simulink library "reorder_library"  (Simulink 6.2)
values from neighbouring files (symbols this model uses):
  bigColBits = 0    [address_gen_dram_mask.m]
  bigRowBits = log2(bigRowLength)    [address_gen_dram_mask.m]
  smallColBits = 0    [address_gen_dram_mask.m]
  smallRowBits = log2(smallRowLength)    [address_gen_dram_mask.m]
undefined symbols (not defined in the file or in its folder): n_bits, order, order_bits
libraries: xbsIndex_r3 x167, fft_library x3, reorder_library x3, xps_library x2, delay_lib x2, simulink x1
settings Model: LastModifiedBy=hchen05

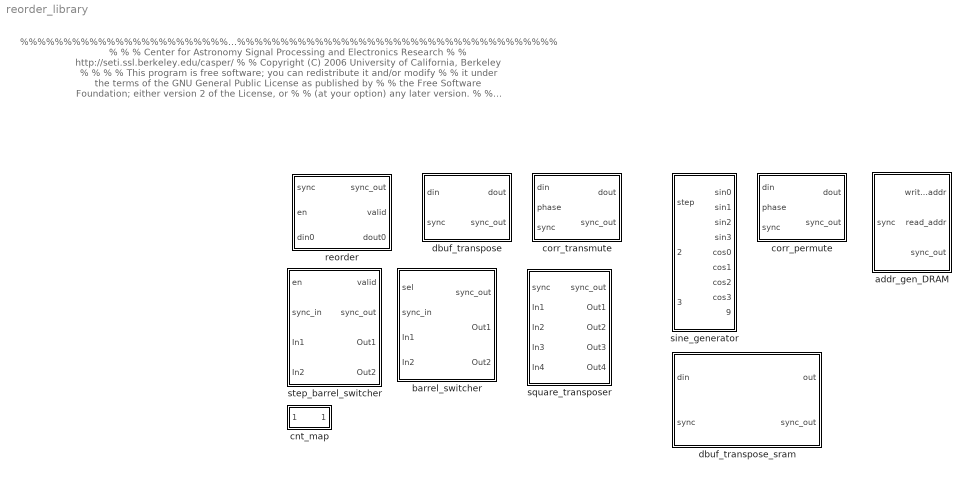
== system reorder_library ==
  note: %%%%%%%%%%%%%%%%%%%%%%%%%%%%%%%%%%%%%%%%%%%%%%%%%%%%%%%%%%%%%%%%%%%%%%%%%%%%%%%
      | %                                                                             %
      | %   Center for Astronomy Signal Processing and Electronics Research           %
      | %   http://seti.ssl.berkeley.edu/casper/                                      %
      | %   Copyright (C) 2006 University of California, Berkeley                     %
      | %                                                                             %
      | %   This program is free software; you can redistribute it and/or modify      %
      | %   it under the terms of the GNU General Public License as published by      %
      | %   the Free Software Foundation; either version 2 of the License, or         %
      | %   (at your option) any later version.                                       %
      | %                                                                             %
      | %   This program is distributed in the hope that it will be useful,           %
      | %   but WITHOUT ANY WARRANTY; without even the implied warranty of            %
      | %   MERCHANTABILITY or FITNESS FOR A PARTICULAR PURPOSE.  See the             %
      | %   GNU General Public License for more details.                              %
      | %                                                                             %
      | %   You should have received a copy of the GNU General Public License along   %
      | %   with this program; if not, write to the Free Software Foundation, Inc.,   %
      | %   51 Franklin Street, Fifth Floor, Boston, MA 02110-1301 USA.               %
      | %                                                                             %
      | %%%%%%%%%%%%%%%%%%%%%%%%%%%%%%%%%%%%%%%%%%%%%%%%%%%%%%%%%%%%%%%%%%%%%%%%%%%%%%%
  addr_gen_DRAM : Subsystem  mask{numSpecs=512, length=1024}
      mask prompts: numSpecs "Number of Spectrums?"; length "Lenght of Spectrum?"
      mask init:
      | address_gen_dram_mask_temp;
  barrel_switcher : Subsystem  mask{n_inputs=1}
      mask prompts: n_inputs "Number of Inputs: (2^?)"
      mask init:
      | barrel_switcher_mask;
  cnt_map : Subsystem  mask(cnt_map){n_bits=2, map=[0 2 1 3], latency=0, old_map=[0 2 1 3]}
      mask prompts: n_bits "Number of bits:"; map "Output order:"; old_map "old map"
      mask init:
      | cnt_map_mask;
  corr_permute : Subsystem  mask{ant_bits=4, add_latency=2, bram_latency=2}
      mask prompts: ant_bits "Number of Antennas: (2^?)"; add_latency "Add Latency"; bram_latency "BRAM Latency"
      mask init:
      | Rows = ant_bits;
  corr_transmute : Subsystem  mask{Rows=2, Cols=3, bram_latency=2, add_latency=2, ant_bits=3}
      mask prompts: Rows "Rows of Matrix (data written in): (2^?)"; Cols "Cols of Matrix (data read out): (2^?)"; bram_latency "BRAM Latency"; add_latency "Add Latency"; ant_bits "Number of Antennas: (2^?)"
  dbuf_transpose : Subsystem  mask{Rows=2, Cols=3, bram_latency=2}
      mask prompts: Rows "Rows of Matrix (data written in): (2^?)"; Cols "Cols of Matrix (data read out): (2^?)"; bram_latency "BRAM Latency"
  dbuf_transpose_sram : Subsystem  mask{length=256, numSpecs=256}
      mask prompts: length "Length of Spectrums"; numSpecs "Number of Spectrums"
      mask help: Sram transpose using double buffering method, maximum size is 256 spectrums by 2048 channels!!
  reorder : Subsystem  mask{map=[0 2 1 3], n_inputs=1, bram_latency=2, map_latency=1}
      mask prompts: map "Output Order:"; n_inputs "Number of inputs"; bram_latency "BRAM Latency"; map_latency "Map Latency"
      mask init:
      | reorder_mask;
  sine_generator : Subsystem  mask{bits=8}
      mask prompts: bits "bitwidth?"
      mask help: Outputs sine and cosine sequences with variable frequency depending on the value of step. If value of step is greater or equal to 2^24 and multiple of 4 then sin0 to sin3 (cos0 to cos3) are consecutive samples of the same sine/cos wave!
  square_transposer : Subsystem  mask{n_inputs=2}
      mask prompts: n_inputs "Number of inputs (2^?):"
      mask init:
      | square_transposer_mask;
  step_barrel_switcher : Subsystem  mask{n_inputs=1, step_dir=Up}
      mask prompts: n_inputs "Number of Inputs: (2^?)"; step_dir "Step Direction"
      mask init:
      | step_barrel_switcher_mask;
      mask StyleString: edit,popup(Up|Down)

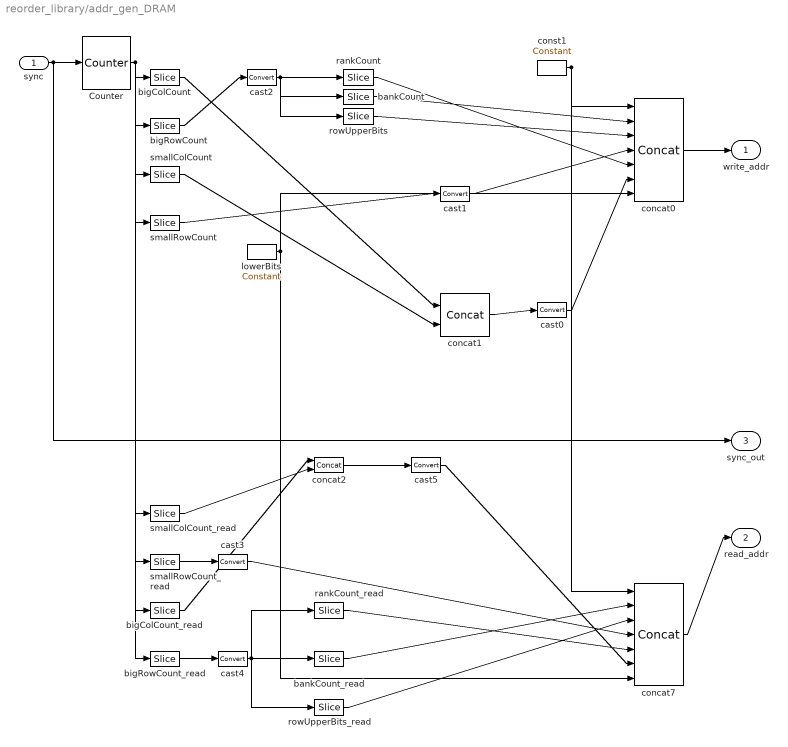
== system reorder_library/addr_gen_DRAM ==
  sync : Inport  Port=1  LatchInput=off
  Counter : xbsIndex_r3/Counter  cnt_type=Free Running  n_bits=counterBitwidth  bin_pt=0  arith_type=Unsigned  start_count=0  cnt_to=Inf  cnt_by_val=1  operation=Up  explicit_period=off  period=1  load_pin=off  rst=on  en=off  dbl_ovrd=off  show_param=off  use_rpm=on  gen_core=off
      settings: xl_area=[0, 0, 0, 0, 0, 0, 0]
  bankCount : xbsIndex_r3/Slice  mode=Upper Bit Location + Width  nbits=2  bit1=-1  base1=MSB of Input  bit0=0  base0=LSB of Input  boolean_output=off  explicit_period=off  period=1  dbl_ovrd=off
  bankCount_read : xbsIndex_r3/Slice  mode=Upper Bit Location + Width  nbits=2  bit1=-1  base1=MSB of Input  bit0=0  base0=LSB of Input  boolean_output=off  explicit_period=off  period=1  dbl_ovrd=off
  bigColCount : xbsIndex_r3/Slice  mode=Lower Bit Location + Width  nbits=bigColBits  bit1=0  base1=MSB of Input  bit0=smallRowBits+smallColBits+8  base0=LSB of Input  boolean_output=off  explicit_period=off  period=1  dbl_ovrd=off
  bigColCount_read : xbsIndex_r3/Slice  mode=Lower Bit Location + Width  nbits=bigColBits  bit1=0  base1=MSB of Input  bit0=bigRowBits  base0=LSB of Input  boolean_output=off  explicit_period=off  period=1  dbl_ovrd=off
  bigRowCount : xbsIndex_r3/Slice  mode=Lower Bit Location + Width  nbits=bigRowBits  bit1=0  base1=MSB of Input  bit0=smallRowBits+smallColBits  base0=LSB of Input  boolean_output=off  explicit_period=off  period=1  dbl_ovrd=off
  bigRowCount_read : xbsIndex_r3/Slice  mode=Lower Bit Location + Width  nbits=bigRowBits  bit1=0  base1=MSB of Input  bit0=0  base0=LSB of Input  boolean_output=off  explicit_period=off  period=1  dbl_ovrd=off
  cast0 : xbsIndex_r3/Convert  arith_type=Unsigned  n_bits=10  bin_pt=0  quantization=Truncate  overflow=Wrap  latency=0  explicit_period=off  period=1  dbl_ovrd=off  show_param=off  inserted_by_tool=off  pipeline=off
      settings: xl_area=[0, 0, 0, 0, 0, 0, 0]
  cast1 : xbsIndex_r3/Convert  arith_type=Unsigned  n_bits=9  bin_pt=0  quantization=Truncate  overflow=Wrap  latency=0  explicit_period=off  period=1  dbl_ovrd=off  show_param=off  inserted_by_tool=off  pipeline=off
      settings: xl_area=[0, 0, 0, 0, 0, 0, 0]
  cast2 : xbsIndex_r3/Convert  arith_type=Unsigned  n_bits=8  bin_pt=0  quantization=Truncate  overflow=Wrap  latency=0  explicit_period=off  period=1  dbl_ovrd=off  show_param=off  inserted_by_tool=off  pipeline=off
      settings: xl_area=[0, 0, 0, 0, 0, 0, 0]
  cast3 : xbsIndex_r3/Convert  arith_type=Unsigned  n_bits=9  bin_pt=0  quantization=Truncate  overflow=Wrap  latency=0  explicit_period=off  period=1  dbl_ovrd=off  show_param=off  inserted_by_tool=off  pipeline=off
      settings: xl_area=[0, 0, 0, 0, 0, 0, 0]
  cast4 : xbsIndex_r3/Convert  arith_type=Unsigned  n_bits=8  bin_pt=0  quantization=Truncate  overflow=Wrap  latency=0  explicit_period=off  period=1  dbl_ovrd=off  show_param=off  inserted_by_tool=off  pipeline=off
      settings: xl_area=[0, 0, 0, 0, 0, 0, 0]
  cast5 : xbsIndex_r3/Convert  arith_type=Unsigned  n_bits=10  bin_pt=0  quantization=Truncate  overflow=Wrap  latency=0  explicit_period=off  period=1  dbl_ovrd=off  show_param=off  inserted_by_tool=off  pipeline=off
      settings: xl_area=[0, 0, 0, 0, 0, 0, 0]
  concat0 : xbsIndex_r3/Concat  num_inputs=7  explicit_period=off  period=1  dbl_ovrd=off
  concat1 : xbsIndex_r3/Concat  num_inputs=2  explicit_period=off  period=1  dbl_ovrd=off
  concat2 : xbsIndex_r3/Concat  num_inputs=2  explicit_period=off  period=1  dbl_ovrd=off
  concat7 : xbsIndex_r3/Concat  num_inputs=7  explicit_period=off  period=1  dbl_ovrd=off
  const1 : xbsIndex_r3/Constant  const=0  equ=P=C  arith_type=Unsigned  n_bits=2  bin_pt=0  opselect=C  inp2=PCIN>>17  opr=+  inp1=P  carry=CIN  iostate=0  explicit_period=on  period=1  dbl_ovrd=off
  lowerBits : xbsIndex_r3/Constant  const=0  equ=P=C  arith_type=Unsigned  n_bits=3  bin_pt=0  opselect=C  inp2=PCIN>>17  opr=+  inp1=P  carry=CIN  iostate=0  explicit_period=on  period=1  dbl_ovrd=off
  rankCount : xbsIndex_r3/Slice  mode=Upper Bit Location + Width  nbits=1  bit1=0  base1=MSB of Input  bit0=0  base0=LSB of Input  boolean_output=off  explicit_period=off  period=1  dbl_ovrd=off
  rankCount_read : xbsIndex_r3/Slice  mode=Upper Bit Location + Width  nbits=1  bit1=0  base1=MSB of Input  bit0=0  base0=LSB of Input  boolean_output=off  explicit_period=off  period=1  dbl_ovrd=off
  rowUpperBits : xbsIndex_r3/Slice  mode=Lower Bit Location + Width  nbits=5  bit1=0  base1=MSB of Input  bit0=0  base0=LSB of Input  boolean_output=off  explicit_period=off  period=1  dbl_ovrd=off
  rowUpperBits_read : xbsIndex_r3/Slice  mode=Lower Bit Location + Width  nbits=5  bit1=0  base1=MSB of Input  bit0=0  base0=LSB of Input  boolean_output=off  explicit_period=off  period=1  dbl_ovrd=off
  smallColCount : xbsIndex_r3/Slice  mode=Lower Bit Location + Width  nbits=smallColBits  bit1=0  base1=MSB of Input  bit0=smallRowBits  base0=LSB of Input  boolean_output=off  explicit_period=off  period=1  dbl_ovrd=off
  smallColCount_read : xbsIndex_r3/Slice  mode=Lower Bit Location + Width  nbits=smallColBits  bit1=0  base1=MSB of Input  bit0=bigRowBits+bigColBits+smallRowBits  base0=LSB of Input  boolean_output=off  explicit_period=off  period=1  dbl_ovrd=off
  smallRowCount : xbsIndex_r3/Slice  mode=Lower Bit Location + Width  nbits=smallRowBits  bit1=0  base1=MSB of Input  bit0=0  base0=LSB of Input  boolean_output=off  explicit_period=off  period=1  dbl_ovrd=off
  smallRowCount_read : xbsIndex_r3/Slice  mode=Lower Bit Location + Width  nbits=smallRowBits  bit1=0  base1=MSB of Input  bit0=bigRowBits+bigColBits  base0=LSB of Input  boolean_output=off  explicit_period=off  period=1  dbl_ovrd=off
  write_addr : Outport
  read_addr : Outport  Port=2
  sync_out : Outport  Port=3
  wires:
  Counter/1 -> bigColCount/1, smallColCount/1, bigColCount_read/1, smallColCount_read/1, smallRowCount/1, bigRowCount/1, smallRowCount_read/1, bigRowCount_read/1
  bigColCount/1 -> concat1/1
  smallColCount/1 -> concat1/2
  concat1/1 -> cast0/1
  smallColCount_read/1 -> concat2/2
  bigColCount_read/1 -> concat2/1
  concat2/1 -> cast5/1
  sync/1 -> Counter/1, sync_out/1
  lowerBits/1 -> concat0/7, concat7/7
  cast0/1 -> concat0/6
  cast5/1 -> concat7/6
  rankCount/1 -> concat0/5
  rankCount_read/1 -> concat7/5
  cast1/1 -> concat0/4
  cast3/1 -> concat7/4
  smallRowCount/1 -> cast1/1
  rowUpperBits/1 -> concat0/3
  rowUpperBits_read/1 -> concat7/3
  bankCount/1 -> concat0/2
  bankCount_read/1 -> concat7/2
  const1/1 -> concat0/1, concat7/1
  bigRowCount/1 -> cast2/1
  cast2/1 -> bankCount/1, rankCount/1, rowUpperBits/1
  smallRowCount_read/1 -> cast3/1
  bigRowCount_read/1 -> cast4/1
  cast4/1 -> rankCount_read/1, bankCount_read/1, rowUpperBits_read/1
  concat0/1 -> write_addr/1
  concat7/1 -> read_addr/1

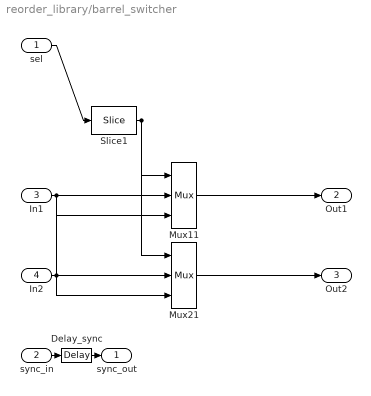
== system reorder_library/barrel_switcher ==
  sel : Inport  Port=1  LatchInput=off
  sync_in : Inport  Port=2  LatchInput=off
  In1 : Inport  Port=3  LatchInput=off
  In2 : Inport  Port=4  LatchInput=off
  Delay_sync : xbsIndex_r3/Delay  latency=1  reg_retiming=off  explicit_period=off  period=1  en=off  accept_only_valid=off  init_zero=on  dbl_ovrd=off  show_param=off
      settings: xl_area=[0, 0, 0, 0, 0, 0, 0]
  Mux11 : xbsIndex_r3/Mux  inputs=2  precision=Full  arith_type="Signed  (2's comp)"  n_bits=8  bin_pt=2  quantization=Truncate  overflow=Wrap  latency=1  explicit_period=off  period=1  en=off  dbl_ovrd=off  show_param=off  mux_type=off  use_rpm=off  gen_core=off
      settings: xl_area=[0, 0, 0, 0, 0, 0, 0]
  Mux21 : xbsIndex_r3/Mux  inputs=2  precision=Full  arith_type="Signed  (2's comp)"  n_bits=8  bin_pt=2  quantization=Truncate  overflow=Wrap  latency=1  explicit_period=off  period=1  en=off  dbl_ovrd=off  show_param=off  mux_type=off  use_rpm=off  gen_core=off
      settings: xl_area=[0, 0, 0, 0, 0, 0, 0]
  Slice1 : xbsIndex_r3/Slice  mode=Upper Bit Location + Width  nbits=1  bit1=-0  base1=MSB of Input  bit0=0  base0=LSB of Input  boolean_output=off  explicit_period=off  period=1  dbl_ovrd=off
  sync_out : Outport
  Out1 : Outport  Port=2
  Out2 : Outport  Port=3
  wires:
  sync_in/1 -> Delay_sync/1
  Delay_sync/1 -> sync_out/1
  sel/1 -> Slice1/1
  Slice1/1 -> Mux11/1, Mux21/1
  In1/1 -> Mux11/2, Mux21/3
  Mux11/1 -> Out1/1
  In2/1 -> Mux21/2, Mux11/3
  Mux21/1 -> Out2/1

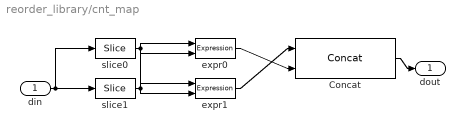
== system reorder_library/cnt_map ==
  din : Inport  Port=1  LatchInput=off
  Concat : xbsIndex_r3/Concat  num_inputs=2  explicit_period=off  period=1  dbl_ovrd=off
  expr0 : xbsIndex_r3/Expression  expression=(in1)|(in0&~in0)|(in1&~in1)  precision=Full  arith_type=Unsigned  n_bits=8  bin_pt=2  align_bp=on  latency=latency  explicit_period=off  period=1  en=off  dbl_ovrd=off  show_param=off
      settings: xl_area=[0, 0, 0, 0, 0, 0, 0]
  expr1 : xbsIndex_r3/Expression  expression=(in0)|(in0&~in0)|(in1&~in1)  precision=Full  arith_type=Unsigned  n_bits=8  bin_pt=2  align_bp=on  latency=latency  explicit_period=off  period=1  en=off  dbl_ovrd=off  show_param=off
      settings: xl_area=[0, 0, 0, 0, 0, 0, 0]
  slice0 : xbsIndex_r3/Slice  mode=Lower Bit Location + Width  nbits=1  bit1=0  base1=MSB of Input  bit0=0  base0=LSB of Input  boolean_output=off  explicit_period=off  period=1  dbl_ovrd=off
  slice1 : xbsIndex_r3/Slice  mode=Lower Bit Location + Width  nbits=1  bit1=-1  base1=MSB of Input  bit0=1  base0=LSB of Input  boolean_output=off  explicit_period=off  period=1  dbl_ovrd=off
  dout : Outport
  wires:
  din/1 -> slice0/1, slice1/1
  slice0/1 -> expr0/1, expr1/1
  slice1/1 -> expr0/2, expr1/2
  expr0/1 -> Concat/2
  expr1/1 -> Concat/1
  Concat/1 -> dout/1

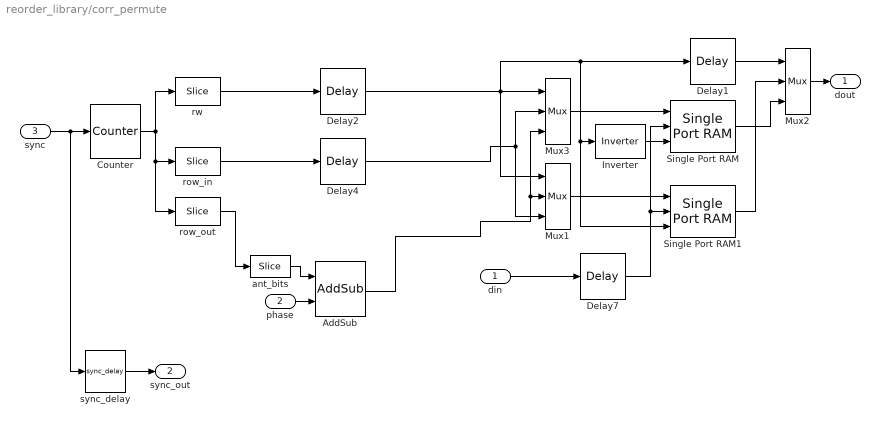
== system reorder_library/corr_permute ==
  din : Inport  Port=1  LatchInput=off
  phase : Inport  Port=2  LatchInput=off
  sync : Inport  Port=3  LatchInput=off
  AddSub : xbsIndex_r3/AddSub  mode=Subtraction  precision=User Defined  arith_type=Unsigned  n_bits=ant_bits  bin_pt=0  quantization=Truncate  overflow=Wrap  latency=add_latency  explicit_period=off  period=1  use_carryin=off  use_carryout=off  en=off  dbl_ovrd=off  show_param=off  use_core=on  pipeline=off  use_rpm=on  gen_core=off
      settings: xl_area=[0, 0, 0, 0, 0, 0, 0]
  Counter : xbsIndex_r3/Counter  cnt_type=Free Running  n_bits="Rows  + 1"  bin_pt=0  arith_type=Unsigned  start_count=0  cnt_to=Inf  cnt_by_val=1  operation=Up  explicit_period=on  period=1  load_pin=off  rst=on  en=off  dbl_ovrd=off  show_param=off  use_rpm=on  gen_core=off
      settings: xl_area=[0, 0, 0, 0, 0, 0, 0]
  Delay1 : xbsIndex_r3/Delay  latency=bram_latency  reg_retiming=off  explicit_period=off  period=1  en=off  accept_only_valid=off  init_zero=on  dbl_ovrd=off  show_param=off
      settings: xl_area=[0, 0, 0, 0, 0, 0, 0]
  Delay2 : xbsIndex_r3/Delay  latency=add_latency  reg_retiming=off  explicit_period=off  period=1  en=off  accept_only_valid=off  init_zero=on  dbl_ovrd=off  show_param=off
      settings: xl_area=[0, 0, 0, 0, 0, 0, 0]
  Delay4 : xbsIndex_r3/Delay  latency=add_latency  reg_retiming=off  explicit_period=off  period=1  en=off  accept_only_valid=off  init_zero=on  dbl_ovrd=off  show_param=off
      settings: xl_area=[0, 0, 0, 0, 0, 0, 0]
  Delay7 : xbsIndex_r3/Delay  latency=add_latency  reg_retiming=off  explicit_period=off  period=1  en=off  accept_only_valid=off  init_zero=on  dbl_ovrd=off  show_param=off
      settings: xl_area=[0, 0, 0, 0, 0, 0, 0]
  Inverter : xbsIndex_r3/Inverter  latency=0  explicit_period=off  period=1  en=off  dbl_ovrd=off  show_param=off
      settings: xl_area=[0, 0, 0, 0, 0, 0, 0]
  Mux1 : xbsIndex_r3/Mux  inputs=2  precision=Full  arith_type="Signed  (2's comp)"  n_bits=8  bin_pt=2  quantization=Truncate  overflow=Wrap  latency=0  explicit_period=off  period=1  en=off  dbl_ovrd=off  show_param=off  mux_type=off  use_rpm=off  gen_core=off
      settings: xl_area=[0, 0, 0, 0, 0, 0, 0]
  Mux2 : xbsIndex_r3/Mux  inputs=2  precision=Full  arith_type="Signed  (2's comp)"  n_bits=8  bin_pt=2  quantization=Truncate  overflow=Wrap  latency=1  explicit_period=off  period=1  en=off  dbl_ovrd=off  show_param=off  mux_type=off  use_rpm=off  gen_core=off
      settings: xl_area=[0, 0, 0, 0, 0, 0, 0]
  Mux3 : xbsIndex_r3/Mux  inputs=2  precision=Full  arith_type="Signed  (2's comp)"  n_bits=8  bin_pt=2  quantization=Truncate  overflow=Wrap  latency=0  explicit_period=off  period=1  en=off  dbl_ovrd=off  show_param=off  mux_type=off  use_rpm=off  gen_core=off
      settings: xl_area=[0, 0, 0, 0, 0, 0, 0]
  Single Port RAM : xbsIndex_r3/Single Port RAM  depth=2^(Rows )  initVector=0  write_mode=Read Before Write  latency=bram_latency  init_zero=on  explicit_period=off  period=1  rst=off  init_reg=0  en=off  dbl_ovrd=off  show_param=off  distributed_mem=off  use_rpm=off  gen_core=off
      settings: xl_area=[0, 0, 0, 0, 0, 0, 0]
  Single Port RAM1 : xbsIndex_r3/Single Port RAM  depth=2^(Rows)  initVector=0  write_mode=Read Before Write  latency=bram_latency  init_zero=on  explicit_period=off  period=1  rst=off  init_reg=0  en=off  dbl_ovrd=off  show_param=off  distributed_mem=off  use_rpm=off  gen_core=off
      settings: xl_area=[0, 0, 0, 0, 0, 0, 0]
  ant_bits : xbsIndex_r3/Slice  mode=Lower Bit Location + Width  nbits=ant_bits  bit1=-1  base1=MSB of Input  bit0=0  base0=LSB of Input  boolean_output=off  explicit_period=off  period=1  dbl_ovrd=off
  row_in : xbsIndex_r3/Slice  mode=Lower Bit Location + Width  nbits=Rows  bit1=0  base1=MSB of Input  bit0=0  base0=LSB of Input  boolean_output=off  explicit_period=off  period=1  dbl_ovrd=off
  row_out : xbsIndex_r3/Slice  mode=Upper Bit Location + Width  nbits=Rows  bit1=-1  base1=MSB of Input  bit0=0  base0=LSB of Input  boolean_output=off  explicit_period=off  period=1  dbl_ovrd=off
  rw : xbsIndex_r3/Slice  mode=Upper Bit Location + Width  nbits=1  bit1=0  base1=MSB of Input  bit0=0  base0=LSB of Input  boolean_output=on  explicit_period=off  period=1  dbl_ovrd=off
  sync_delay : fft_library/sync_delay  DelayLen=2^Rows+ add_latency + bram_latency + 1
  dout : Outport
  sync_out : Outport  Port=2
  wires:
  AddSub/1 -> Mux1/2, Mux3/3
  Inverter/1 -> Single Port RAM/3
  Mux2/1 -> dout/1
  Delay1/1 -> Mux2/1
  din/1 -> Delay7/1
  Single Port RAM/1 -> Mux2/3
  Single Port RAM1/1 -> Mux2/2
  Mux1/1 -> Single Port RAM1/1
  Mux3/1 -> Single Port RAM/1
  sync/1 -> sync_delay/1, Counter/1
  row_in/1 -> Delay4/1
  rw/1 -> Delay2/1
  Counter/1 -> row_out/1, row_in/1, rw/1
  sync_delay/1 -> sync_out/1
  phase/1 -> AddSub/2
  ant_bits/1 -> AddSub/1
  Delay2/1 -> Single Port RAM1/3, Inverter/1, Delay1/1, Mux1/1, Mux3/1
  Delay4/1 -> Mux1/3, Mux3/2
  row_out/1 -> ant_bits/1
  Delay7/1 -> Single Port RAM/2, Single Port RAM1/2

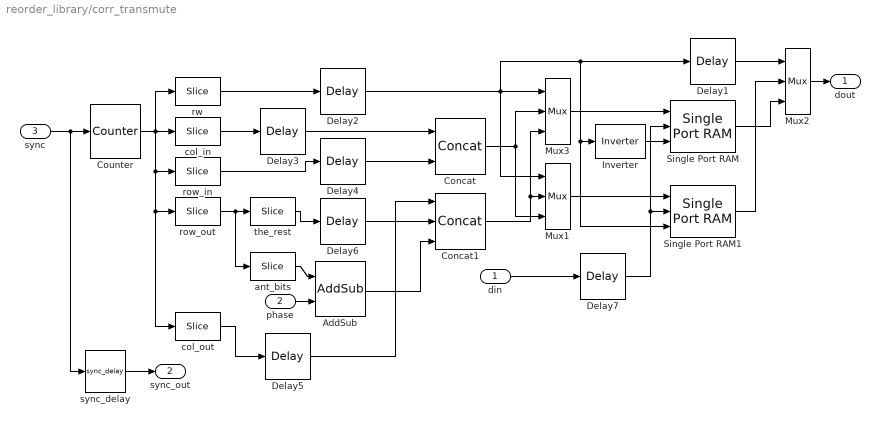
== system reorder_library/corr_transmute ==
  din : Inport  Port=1  LatchInput=off
  phase : Inport  Port=2  LatchInput=off
  sync : Inport  Port=3  LatchInput=off
  AddSub : xbsIndex_r3/AddSub  mode=Addition  precision=User Defined  arith_type=Unsigned  n_bits=ant_bits  bin_pt=0  quantization=Truncate  overflow=Wrap  latency=add_latency  explicit_period=off  period=1  use_carryin=off  use_carryout=off  en=off  dbl_ovrd=off  show_param=off  use_core=on  pipeline=off  use_rpm=on  gen_core=off
      settings: xl_area=[0, 0, 0, 0, 0, 0, 0]
  Concat : xbsIndex_r3/Concat  num_inputs=2  explicit_period=off  period=1  dbl_ovrd=off
  Concat1 : xbsIndex_r3/Concat  num_inputs=3  explicit_period=off  period=1  dbl_ovrd=off
  Counter : xbsIndex_r3/Counter  cnt_type=Free Running  n_bits=Rows + Cols + 1  bin_pt=0  arith_type=Unsigned  start_count=0  cnt_to=Inf  cnt_by_val=1  operation=Up  explicit_period=on  period=1  load_pin=off  rst=on  en=off  dbl_ovrd=off  show_param=off  use_rpm=on  gen_core=off
      settings: xl_area=[0, 0, 0, 0, 0, 0, 0]
  Delay1 : xbsIndex_r3/Delay  latency=bram_latency  reg_retiming=off  explicit_period=off  period=1  en=off  accept_only_valid=off  init_zero=on  dbl_ovrd=off  show_param=off
      settings: xl_area=[0, 0, 0, 0, 0, 0, 0]
  Delay{2..7} (6 alike) : xbsIndex_r3/Delay  latency=add_latency  reg_retiming=off  explicit_period=off  period=1  en=off  accept_only_valid=off  init_zero=on  dbl_ovrd=off  show_param=off
      settings: xl_area=[0, 0, 0, 0, 0, 0, 0]
  Inverter : xbsIndex_r3/Inverter  latency=0  explicit_period=off  period=1  en=off  dbl_ovrd=off  show_param=off
      settings: xl_area=[0, 0, 0, 0, 0, 0, 0]
  Mux1 : xbsIndex_r3/Mux  inputs=2  precision=Full  arith_type="Signed  (2's comp)"  n_bits=8  bin_pt=2  quantization=Truncate  overflow=Wrap  latency=0  explicit_period=off  period=1  en=off  dbl_ovrd=off  show_param=off  mux_type=off  use_rpm=off  gen_core=off
      settings: xl_area=[0, 0, 0, 0, 0, 0, 0]
  Mux2 : xbsIndex_r3/Mux  inputs=2  precision=Full  arith_type="Signed  (2's comp)"  n_bits=8  bin_pt=2  quantization=Truncate  overflow=Wrap  latency=1  explicit_period=off  period=1  en=off  dbl_ovrd=off  show_param=off  mux_type=off  use_rpm=off  gen_core=off
      settings: xl_area=[0, 0, 0, 0, 0, 0, 0]
  Mux3 : xbsIndex_r3/Mux  inputs=2  precision=Full  arith_type="Signed  (2's comp)"  n_bits=8  bin_pt=2  quantization=Truncate  overflow=Wrap  latency=0  explicit_period=off  period=1  en=off  dbl_ovrd=off  show_param=off  mux_type=off  use_rpm=off  gen_core=off
      settings: xl_area=[0, 0, 0, 0, 0, 0, 0]
  Single Port RAM : xbsIndex_r3/Single Port RAM  depth=2^(Rows + Cols)  initVector=0  write_mode=Read Before Write  latency=bram_latency  init_zero=on  explicit_period=off  period=1  rst=off  init_reg=0  en=off  dbl_ovrd=off  show_param=off  distributed_mem=off  use_rpm=off  gen_core=off
      settings: xl_area=[0, 0, 0, 0, 0, 0, 0]
  Single Port RAM1 : xbsIndex_r3/Single Port RAM  depth=2^(Rows + Cols)  initVector=0  write_mode=Read Before Write  latency=bram_latency  init_zero=on  explicit_period=off  period=1  rst=off  init_reg=0  en=off  dbl_ovrd=off  show_param=off  distributed_mem=off  use_rpm=off  gen_core=off
      settings: xl_area=[0, 0, 0, 0, 0, 0, 0]
  ant_bits : xbsIndex_r3/Slice  mode=Lower Bit Location + Width  nbits=ant_bits  bit1=-1  base1=MSB of Input  bit0=0  base0=LSB of Input  boolean_output=off  explicit_period=off  period=1  dbl_ovrd=off
  col_in : xbsIndex_r3/Slice  mode=Upper Bit Location + Width  nbits=Cols  bit1=-1  base1=MSB of Input  bit0=0  base0=LSB of Input  boolean_output=off  explicit_period=off  period=1  dbl_ovrd=off
  col_out : xbsIndex_r3/Slice  mode=Lower Bit Location + Width  nbits=Cols  bit1=-1  base1=MSB of Input  bit0=0  base0=LSB of Input  boolean_output=off  explicit_period=off  period=1  dbl_ovrd=off
  row_in : xbsIndex_r3/Slice  mode=Lower Bit Location + Width  nbits=Rows  bit1=0  base1=MSB of Input  bit0=0  base0=LSB of Input  boolean_output=off  explicit_period=off  period=1  dbl_ovrd=off
  row_out : xbsIndex_r3/Slice  mode=Upper Bit Location + Width  nbits=Rows  bit1=-1  base1=MSB of Input  bit0=0  base0=LSB of Input  boolean_output=off  explicit_period=off  period=1  dbl_ovrd=off
  rw : xbsIndex_r3/Slice  mode=Upper Bit Location + Width  nbits=1  bit1=0  base1=MSB of Input  bit0=0  base0=LSB of Input  boolean_output=on  explicit_period=off  period=1  dbl_ovrd=off
  sync_delay : fft_library/sync_delay  DelayLen=2^(Rows + Cols) + add_latency + bram_latency + 1
  the_rest : xbsIndex_r3/Slice  mode=Two Bit Locations  nbits=Cols  bit1=0  base1=MSB of Input  bit0=ant_bits  base0=LSB of Input  boolean_output=off  explicit_period=off  period=1  dbl_ovrd=off
  dout : Outport
  sync_out : Outport  Port=2
  wires:
  Inverter/1 -> Single Port RAM/3
  Mux2/1 -> dout/1
  Delay1/1 -> Mux2/1
  din/1 -> Delay7/1
  Single Port RAM/1 -> Mux2/3
  Single Port RAM1/1 -> Mux2/2
  Mux1/1 -> Single Port RAM1/1
  Mux3/1 -> Single Port RAM/1
  sync/1 -> sync_delay/1, Counter/1
  row_in/1 -> Delay4/1
  col_in/1 -> Delay3/1
  Concat1/1 -> Mux1/2, Mux3/3
  Concat/1 -> Mux1/3, Mux3/2
  rw/1 -> Delay2/1
  Counter/1 -> row_out/1, col_out/1, row_in/1, col_in/1, rw/1
  sync_delay/1 -> sync_out/1
  phase/1 -> AddSub/2
  ant_bits/1 -> AddSub/1
  Delay2/1 -> Single Port RAM1/3, Inverter/1, Delay1/1, Mux1/1, Mux3/1
  Delay3/1 -> Concat/1
  Delay4/1 -> Concat/2
  the_rest/1 -> Delay6/1
  row_out/1 -> the_rest/1, ant_bits/1
  col_out/1 -> Delay5/1
  Delay5/1 -> Concat1/1
  Delay6/1 -> Concat1/2
  AddSub/1 -> Concat1/3
  Delay7/1 -> Single Port RAM/2, Single Port RAM1/2

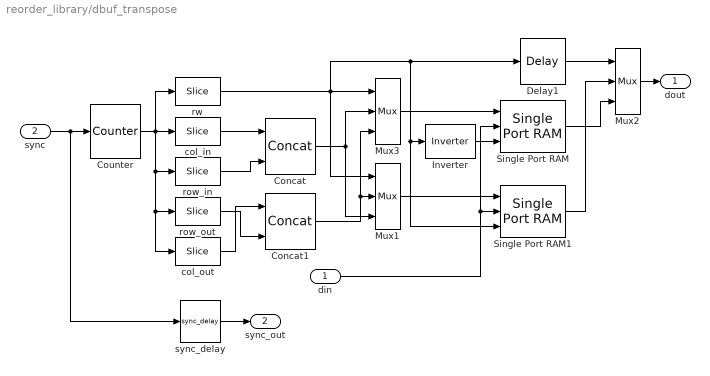
== system reorder_library/dbuf_transpose ==
  din : Inport  Port=1  LatchInput=off
  sync : Inport  Port=2  LatchInput=off
  Concat : xbsIndex_r3/Concat  num_inputs=2  explicit_period=off  period=1  dbl_ovrd=off
  Concat1 : xbsIndex_r3/Concat  num_inputs=2  explicit_period=off  period=1  dbl_ovrd=off
  Counter : xbsIndex_r3/Counter  cnt_type=Free Running  n_bits=Rows + Cols + 1  bin_pt=0  arith_type=Unsigned  start_count=0  cnt_to=Inf  cnt_by_val=1  operation=Up  explicit_period=on  period=1  load_pin=off  rst=on  en=off  dbl_ovrd=off  show_param=off  use_rpm=on  gen_core=off
      settings: xl_area=[0, 0, 0, 0, 0, 0, 0]
  Delay1 : xbsIndex_r3/Delay  latency=bram_latency  reg_retiming=off  explicit_period=off  period=1  en=off  accept_only_valid=off  init_zero=on  dbl_ovrd=off  show_param=off
      settings: xl_area=[0, 0, 0, 0, 0, 0, 0]
  Inverter : xbsIndex_r3/Inverter  latency=0  explicit_period=off  period=1  en=off  dbl_ovrd=off  show_param=off
      settings: xl_area=[0, 0, 0, 0, 0, 0, 0]
  Mux1 : xbsIndex_r3/Mux  inputs=2  precision=Full  arith_type="Signed  (2's comp)"  n_bits=8  bin_pt=2  quantization=Truncate  overflow=Wrap  latency=0  explicit_period=off  period=1  en=off  dbl_ovrd=off  show_param=off  mux_type=off  use_rpm=off  gen_core=off
      settings: xl_area=[0, 0, 0, 0, 0, 0, 0]
  Mux2 : xbsIndex_r3/Mux  inputs=2  precision=Full  arith_type="Signed  (2's comp)"  n_bits=8  bin_pt=2  quantization=Truncate  overflow=Wrap  latency=1  explicit_period=off  period=1  en=off  dbl_ovrd=off  show_param=off  mux_type=off  use_rpm=off  gen_core=off
      settings: xl_area=[0, 0, 0, 0, 0, 0, 0]
  Mux3 : xbsIndex_r3/Mux  inputs=2  precision=Full  arith_type="Signed  (2's comp)"  n_bits=8  bin_pt=2  quantization=Truncate  overflow=Wrap  latency=0  explicit_period=off  period=1  en=off  dbl_ovrd=off  show_param=off  mux_type=off  use_rpm=off  gen_core=off
      settings: xl_area=[0, 0, 0, 0, 0, 0, 0]
  Single Port RAM : xbsIndex_r3/Single Port RAM  depth=2^(Rows + Cols)  initVector=0  write_mode=Read Before Write  latency=bram_latency  init_zero=on  explicit_period=off  period=1  rst=off  init_reg=0  en=off  dbl_ovrd=off  show_param=off  distributed_mem=off  use_rpm=off  gen_core=off
      settings: xl_area=[0, 0, 0, 0, 0, 0, 0]
  Single Port RAM1 : xbsIndex_r3/Single Port RAM  depth=2^(Rows + Cols)  initVector=0  write_mode=Read Before Write  latency=bram_latency  init_zero=on  explicit_period=off  period=1  rst=off  init_reg=0  en=off  dbl_ovrd=off  show_param=off  distributed_mem=off  use_rpm=off  gen_core=off
      settings: xl_area=[0, 0, 0, 0, 0, 0, 0]
  col_in : xbsIndex_r3/Slice  mode=Upper Bit Location + Width  nbits=Cols  bit1=-1  base1=MSB of Input  bit0=0  base0=LSB of Input  boolean_output=off  explicit_period=off  period=1  dbl_ovrd=off
  col_out : xbsIndex_r3/Slice  mode=Lower Bit Location + Width  nbits=Cols  bit1=-1  base1=MSB of Input  bit0=0  base0=LSB of Input  boolean_output=off  explicit_period=off  period=1  dbl_ovrd=off
  row_in : xbsIndex_r3/Slice  mode=Lower Bit Location + Width  nbits=Rows  bit1=0  base1=MSB of Input  bit0=0  base0=LSB of Input  boolean_output=off  explicit_period=off  period=1  dbl_ovrd=off
  row_out : xbsIndex_r3/Slice  mode=Upper Bit Location + Width  nbits=Rows  bit1=-1  base1=MSB of Input  bit0=0  base0=LSB of Input  boolean_output=off  explicit_period=off  period=1  dbl_ovrd=off
  rw : xbsIndex_r3/Slice  mode=Upper Bit Location + Width  nbits=1  bit1=0  base1=MSB of Input  bit0=0  base0=LSB of Input  boolean_output=on  explicit_period=off  period=1  dbl_ovrd=off
  sync_delay : fft_library/sync_delay  DelayLen=2^(Rows + Cols) + bram_latency + 1
  dout : Outport
  sync_out : Outport  Port=2
  wires:
  sync_delay/1 -> sync_out/1
  Counter/1 -> rw/1, col_in/1, row_in/1, col_out/1, row_out/1
  rw/1 -> Mux3/1, Mux1/1, Delay1/1, Inverter/1, Single Port RAM1/3
  Concat/1 -> Mux3/2, Mux1/3
  Concat1/1 -> Mux3/3, Mux1/2
  col_in/1 -> Concat/1
  row_in/1 -> Concat/2
  sync/1 -> Counter/1, sync_delay/1
  Mux3/1 -> Single Port RAM/1
  Mux1/1 -> Single Port RAM1/1
  Single Port RAM1/1 -> Mux2/2
  Single Port RAM/1 -> Mux2/3
  din/1 -> Single Port RAM1/2, Single Port RAM/2
  Delay1/1 -> Mux2/1
  Mux2/1 -> dout/1
  Inverter/1 -> Single Port RAM/3
  col_out/1 -> Concat1/1
  row_out/1 -> Concat1/2

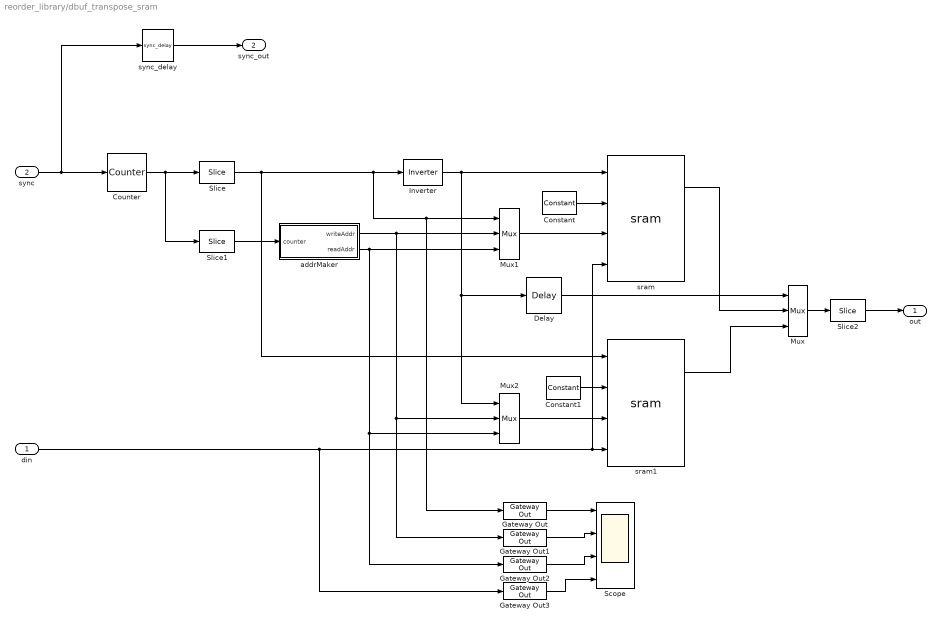
== system reorder_library/dbuf_transpose_sram ==
  din : Inport  Port=1  LatchInput=off
  "sync\t" : Inport  Port=2  LatchInput=off
  Constant : xbsIndex_r3/Constant  const=15  equ=P=C  arith_type=Unsigned  n_bits=4  bin_pt=0  opselect=C  inp2=PCIN>>17  opr=+  inp1=P  carry=CIN  iostate=0  explicit_period=on  period=1  dbl_ovrd=off
  Constant1 : xbsIndex_r3/Constant  const=15  equ=P=C  arith_type=Unsigned  n_bits=4  bin_pt=0  opselect=C  inp2=PCIN>>17  opr=+  inp1=P  carry=CIN  iostate=0  explicit_period=on  period=1  dbl_ovrd=off
  Counter : xbsIndex_r3/Counter  cnt_type=Free Running  n_bits=log2(length)+log2(numSpecs)+1  bin_pt=0  arith_type=Unsigned  start_count=0  cnt_to=Inf  cnt_by_val=1  operation=Up  explicit_period=off  period=1  load_pin=off  rst=on  en=off  dbl_ovrd=off  show_param=off  use_rpm=on  gen_core=off
      settings: xl_area=[0, 0, 0, 0, 0, 0, 0]
  Delay : xbsIndex_r3/Delay  latency=4  reg_retiming=off  explicit_period=off  period=1  en=off  accept_only_valid=off  init_zero=on  dbl_ovrd=off  show_param=off
      settings: xl_area=[0, 0, 0, 0, 0, 0, 0]
  Gateway Out{,1..3} (4 alike) : xbsIndex_r3/Gateway Out  output_type=Double  nbits=8  bin_pt=6  arith_type=Boolean  quantization=Truncate  overflow=Wrap  hdl_port=off  timing_constraint=None  locs_specified=off  LOCs={}  needs_fixed_name=off  show_param=off
      settings: xl_area=[0, 0, 0, 0, 0, 0, 0]
  Inverter : xbsIndex_r3/Inverter  latency=0  explicit_period=off  period=1  en=off  dbl_ovrd=off  show_param=off
      settings: xl_area=[0, 0, 0, 0, 0, 0, 0]
  Mux : xbsIndex_r3/Mux  inputs=2  precision=Full  arith_type="Signed  (2's comp)"  n_bits=8  bin_pt=2  quantization=Truncate  overflow=Wrap  latency=0  explicit_period=off  period=1  en=off  dbl_ovrd=off  show_param=off  mux_type=off  use_rpm=off  gen_core=off
      settings: xl_area=[0, 0, 0, 0, 0, 0, 0]
  Mux1 : xbsIndex_r3/Mux  inputs=2  precision=Full  arith_type="Signed  (2's comp)"  n_bits=8  bin_pt=2  quantization=Truncate  overflow=Wrap  latency=0  explicit_period=off  period=1  en=off  dbl_ovrd=off  show_param=off  mux_type=off  use_rpm=off  gen_core=off
      settings: xl_area=[0, 0, 0, 0, 0, 0, 0]
  Mux2 : xbsIndex_r3/Mux  inputs=2  precision=Full  arith_type="Signed  (2's comp)"  n_bits=8  bin_pt=2  quantization=Truncate  overflow=Wrap  latency=0  explicit_period=off  period=1  en=off  dbl_ovrd=off  show_param=off  mux_type=off  use_rpm=off  gen_core=off
      settings: xl_area=[0, 0, 0, 0, 0, 0, 0]
  Scope : Scope  NumInputPorts=4
      settings: YMin=-5~-5~-5~-5  YMax=5~5~5~5  SaveName=ScopeData2
  Slice : xbsIndex_r3/Slice  mode=Upper Bit Location + Width  nbits=1  bit1=0  base1=MSB of Input  bit0=0  base0=LSB of Input  boolean_output=off  explicit_period=off  period=1  dbl_ovrd=off
  Slice1 : xbsIndex_r3/Slice  mode=Lower Bit Location + Width  nbits=log2(length)+log2(numSpecs)  bit1=0  base1=MSB of Input  bit0=0  base0=LSB of Input  boolean_output=off  explicit_period=off  period=1  dbl_ovrd=off
  Slice2 : xbsIndex_r3/Slice  mode=Lower Bit Location + Width  nbits=32  bit1=0  base1=MSB of Input  bit0=0  base0=LSB of Input  boolean_output=off  explicit_period=off  period=1  dbl_ovrd=off
  addrMaker : Subsystem  mask{length=length, numSpecs=numSpecs}
      mask prompts: length "Spectrum Lenght"; numSpecs "Number of Spectrums"
  sram : xps_library/sram  Tag=xps:sram  sram=0  arith_type=Unsigned  bin_pt=0  sample_period=1  use_sim=on
  sram1 : xps_library/sram  Tag=xps:sram  sram=1  arith_type=Unsigned  bin_pt=0  sample_period=1  use_sim=on
  sync_delay : delay_lib/sync_delay  DelayLen=length*numSpecs+4
      link override Constant: equ=P=C
      link override Constant1: equ=P=C
      link override Constant2: equ=P=C
      link override Constant3: equ=P=C
  out : Outport
  sync_out : Outport  Port=2
  wires:
  Slice2/1 -> out/1
  Delay/1 -> Mux/1
  Gateway Out3/1 -> Scope/4
  Gateway Out2/1 -> Scope/3
  Gateway Out1/1 -> Scope/2
  Gateway Out/1 -> Scope/1
  sram1/1 -> Mux/3
  sync_delay/1 -> sync_out/1
  addrMaker/2(readAddr) -> Mux2/3, Gateway Out2/1, Mux1/3
  addrMaker/1(writeAddr) -> Gateway Out1/1, Mux2/2, Mux1/2
  Constant1/1 -> sram1/2
  Constant/1 -> sram/2
  Mux2/1 -> sram1/3
  Mux1/1 -> sram/3
  sram/1 -> Mux/2
  Mux/1 -> Slice2/1
  din/1 -> Gateway Out3/1, sram/4, sram1/4
  Slice1/1 -> addrMaker/1(counter)
  Inverter/1 -> Delay/1, Mux2/1, sram/1
  Slice/1 -> Gateway Out/1, Mux1/1, Inverter/1, sram1/1
  Counter/1 -> Slice1/1, Slice/1
  "sync\t"/1 -> sync_delay/1, Counter/1

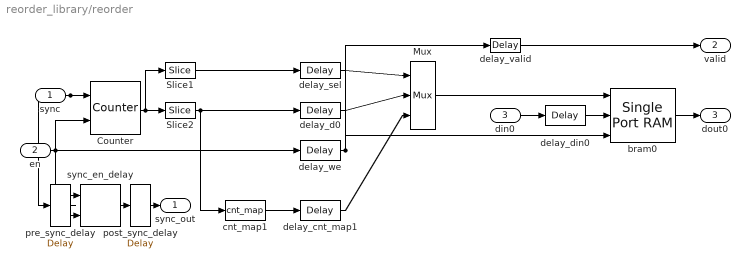
== system reorder_library/reorder ==
  sync : Inport  Port=1  LatchInput=off
  en : Inport  Port=2  LatchInput=off
  din0 : Inport  Port=3  LatchInput=off
  Counter : xbsIndex_r3/Counter  cnt_type=Count Limited  n_bits=n_bits + order_bits  bin_pt=0  arith_type=Unsigned  start_count=0  cnt_to=2^n_bits * order - 1  cnt_by_val=1  operation=Up  explicit_period=off  period=1  load_pin=off  rst=on  en=on  dbl_ovrd=off  show_param=off  use_rpm=on  gen_core=off
      settings: xl_area=[0, 0, 0, 0, 0, 0, 0]
  Mux : xbsIndex_r3/Mux  inputs=2  precision=Full  arith_type="Signed  (2's comp)"  n_bits=8  bin_pt=2  quantization=Truncate  overflow=Wrap  latency=1  explicit_period=off  period=1  en=off  dbl_ovrd=off  show_param=off  mux_type=off  use_rpm=off  gen_core=off
      settings: xl_area=[0, 0, 0, 0, 0, 0, 0]
  Slice1 : xbsIndex_r3/Slice  mode=Upper Bit Location + Width  nbits=order_bits  bit1=0  base1=MSB of Input  bit0=0  base0=LSB of Input  boolean_output=off  explicit_period=off  period=1  dbl_ovrd=off
  Slice2 : xbsIndex_r3/Slice  mode=Lower Bit Location + Width  nbits=n_bits  bit1=0  base1=MSB of Input  bit0=0  base0=LSB of Input  boolean_output=off  explicit_period=off  period=1  dbl_ovrd=off
  bram0 : xbsIndex_r3/Single Port RAM  depth=2^n_bits  initVector=sin(pi*(0:15)/16)  write_mode=Read Before Write  latency=bram_latency  init_zero=on  explicit_period=off  period=1  rst=off  init_reg=0  en=off  dbl_ovrd=off  show_param=off  distributed_mem=off  use_rpm=off  gen_core=off
      settings: xl_area=[0, 0, 0, 0, 0, 0, 0]
  cnt_map1 : reorder_library/cnt_map  n_bits=n_bits  map=map  latency=map_latency  old_map=[0 2 1 3]
  delay_cnt_map1 : xbsIndex_r3/Delay  latency=0*map_latency  reg_retiming=off  explicit_period=off  period=1  en=off  accept_only_valid=off  init_zero=on  dbl_ovrd=off  show_param=off
      settings: xl_area=[0, 0, 0, 0, 0, 0, 0]
  delay_d0 : xbsIndex_r3/Delay  latency=(order-1)*map_latency  reg_retiming=off  explicit_period=off  period=1  en=off  accept_only_valid=off  init_zero=on  dbl_ovrd=off  show_param=off
      settings: xl_area=[0, 0, 0, 0, 0, 0, 0]
  delay_din0 : xbsIndex_r3/Delay  latency=(order-1)*map_latency+1  reg_retiming=off  explicit_period=off  period=1  en=off  accept_only_valid=off  init_zero=on  dbl_ovrd=off  show_param=off
      settings: xl_area=[0, 0, 0, 0, 0, 0, 0]
  delay_sel : xbsIndex_r3/Delay  latency=(order-1)*map_latency  reg_retiming=off  explicit_period=off  period=1  en=off  accept_only_valid=off  init_zero=on  dbl_ovrd=off  show_param=off
      settings: xl_area=[0, 0, 0, 0, 0, 0, 0]
  delay_valid : xbsIndex_r3/Delay  latency=bram_latency+1  reg_retiming=off  explicit_period=off  period=1  en=off  accept_only_valid=off  init_zero=on  dbl_ovrd=off  show_param=off
      settings: xl_area=[0, 0, 0, 0, 0, 0, 0]
  delay_we : xbsIndex_r3/Delay  latency=(order-1)*map_latency  reg_retiming=off  explicit_period=off  period=1  en=off  accept_only_valid=off  init_zero=on  dbl_ovrd=off  show_param=off
      settings: xl_area=[0, 0, 0, 0, 0, 0, 0]
  post_sync_delay : xbsIndex_r3/Delay  latency=bram_latency+1  reg_retiming=off  explicit_period=off  period=1  en=off  accept_only_valid=off  init_zero=on  dbl_ovrd=off  show_param=off
      settings: xl_area=[0, 0, 0, 0, 0, 0, 0]
  pre_sync_delay : xbsIndex_r3/Delay  latency=(order-1)*map_latency  reg_retiming=off  explicit_period=off  period=1  en=off  accept_only_valid=off  init_zero=on  dbl_ovrd=off  show_param=off
      settings: xl_area=[0, 0, 0, 0, 0, 0, 0]
  sync_en_delay : delay_lib/sync_en_delay  DelayLen=length(map)
  sync_out : Outport
  valid : Outport  Port=2
  dout0 : Outport  Port=3
  wires:
  sync/1 -> Counter/1, pre_sync_delay/1
  en/1 -> Counter/2, sync_en_delay/2, delay_we/1
  Counter/1 -> Slice1/1, Slice2/1
  Slice1/1 -> delay_sel/1
  delay_sel/1 -> Mux/1
  Slice2/1 -> delay_d0/1, cnt_map1/1
  delay_d0/1 -> Mux/2
  pre_sync_delay/1 -> sync_en_delay/1
  sync_en_delay/1 -> post_sync_delay/1
  post_sync_delay/1 -> sync_out/1
  delay_we/1 -> delay_valid/1, bram0/3
  delay_valid/1 -> valid/1
  Mux/1 -> bram0/1
  din0/1 -> delay_din0/1
  delay_din0/1 -> bram0/2
  bram0/1 -> dout0/1
  cnt_map1/1 -> delay_cnt_map1/1
  delay_cnt_map1/1 -> Mux/3

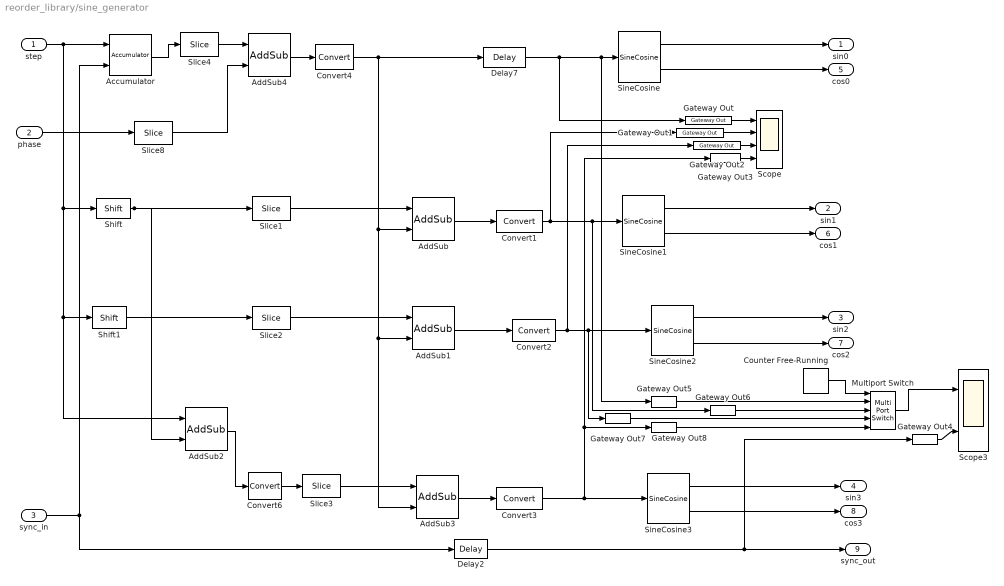
== system reorder_library/sine_generator ==
  step : Inport  Port=1  LatchInput=off
  phase : Inport  Port=2  LatchInput=off
  sync_in : Inport  Port=3  LatchInput=off
  Accumulator : xbsIndex_r3/Accumulator  n_bits=32  overflow=Wrap  operation=Add  scale=1  explicit_period=off  period=1  rst=on  hasbypass=off  en=off  dbl_ovrd=off  show_param=off  gen_core=off  use_rpm=on
      settings: xl_area=[0, 0, 0, 0, 0, 0, 0]
  AddSub{,1,3..4} (4 alike) : xbsIndex_r3/AddSub  mode=Addition  precision=Full  arith_type=Unsigned  n_bits=10  bin_pt=0  quantization="Round  (unbiased: +/- Inf)"  overflow=Wrap  latency=2  explicit_period=off  period=1  use_carryin=off  use_carryout=off  en=off  dbl_ovrd=off  show_param=off  use_core=on  pipeline=on  use_rpm=on  gen_core=off
      settings: xl_area=[0, 0, 0, 0, 0, 0, 0]
  AddSub2 : xbsIndex_r3/AddSub  mode=Subtraction  precision=Full  arith_type=Unsigned  n_bits=10  bin_pt=0  quantization="Round  (unbiased: +/- Inf)"  overflow=Wrap  latency=2  explicit_period=off  period=1  use_carryin=off  use_carryout=off  en=off  dbl_ovrd=off  show_param=off  use_core=on  pipeline=on  use_rpm=on  gen_core=off
      settings: xl_area=[0, 0, 0, 0, 0, 0, 0]
  Convert{1..4} (4 alike) : xbsIndex_r3/Convert  arith_type=Unsigned  n_bits=10  bin_pt=0  quantization="Round  (unbiased: Even Values)"  overflow=Wrap  latency=2  explicit_period=off  period=1  dbl_ovrd=off  show_param=off  inserted_by_tool=off  pipeline=off
      settings: xl_area=[0, 0, 0, 0, 0, 0, 0]
  Convert6 : xbsIndex_r3/Convert  arith_type=Unsigned  n_bits=32  bin_pt=0  quantization="Round  (unbiased: Even Values)"  overflow=Wrap  latency=2  explicit_period=off  period=1  dbl_ovrd=off  show_param=off  inserted_by_tool=off  pipeline=off
      settings: xl_area=[0, 0, 0, 0, 0, 0, 0]
  Counter Free-Running : simulink/Sources/Counter Free-Running  NumBits=2  tsamp=.25
  Delay2 : xbsIndex_r3/Delay  latency=10  reg_retiming=off  explicit_period=off  period=1  en=off  accept_only_valid=off  init_zero=on  dbl_ovrd=off  show_param=off
      settings: xl_area=[0, 0, 0, 0, 0, 0, 0]
  Delay7 : xbsIndex_r3/Delay  latency=4  reg_retiming=off  explicit_period=off  period=1  en=off  accept_only_valid=off  init_zero=on  dbl_ovrd=off  show_param=off
      settings: xl_area=[0, 0, 0, 0, 0, 0, 0]
  Gateway Out{,1..8} (9 alike) : xbsIndex_r3/Gateway Out  output_type=Double  nbits=8  bin_pt=6  arith_type=Boolean  quantization=Truncate  overflow=Wrap  hdl_port=off  timing_constraint=None  locs_specified=off  LOCs={}  needs_fixed_name=off  show_param=off
      settings: xl_area=[0, 0, 0, 0, 0, 0, 0]
  Multiport Switch : MultiPortSwitch  zeroidx=on
  Scope : Scope  NumInputPorts=4
      settings: YMin=-5~-5~-5~-5  YMax=5~5~5~5  SaveName=ScopeData3
  Scope3 : Scope  NumInputPorts=2
      settings: YMin=-5~-5  YMax=5~5  SaveName=ScopeData4
  Shift : xbsIndex_r3/Shift  shift_dir=Right  shift_bits=2  precision=Full  arith_type="Signed  (2's comp)"  n_bits=8  bin_pt=2  quantization=Truncate  overflow=Wrap  latency=0  explicit_period=off  period=1  en=off  dbl_ovrd=off  show_param=off
      settings: xl_area=[0, 0, 0, 0, 0, 0, 0]
  Shift1 : xbsIndex_r3/Shift  shift_dir=Right  shift_bits=1  precision=Full  arith_type="Signed  (2's comp)"  n_bits=8  bin_pt=2  quantization=Truncate  overflow=Wrap  latency=0  explicit_period=off  period=1  en=off  dbl_ovrd=off  show_param=off
      settings: xl_area=[0, 0, 0, 0, 0, 0, 0]
  SineCosine{,1..3} (4 alike) : xbsIndex_r3/SineCosine  mode=Sine and Cosine  neg_sin=off  neg_cos=off  n_bits=bits  latency=2  sym_output=off  explicit_period=off  period=1  en=off  dbl_ovrd=off  show_param=off  mem_type=Block RAM  pipeline=on  use_rpm=on  gen_core=off
      settings: xl_area=[0, 0, 0, 0, 0, 0, 0]
  Slice{1..4} (4 alike) : xbsIndex_r3/Slice  mode=Upper Bit Location + Width  nbits=10  bit1=-2  base1=MSB of Input  bit0=0  base0=LSB of Input  boolean_output=off  explicit_period=off  period=1  dbl_ovrd=off
  Slice8 : xbsIndex_r3/Slice  mode=Lower Bit Location + Width  nbits=10  bit1=0  base1=MSB of Input  bit0=0  base0=LSB of Input  boolean_output=off  explicit_period=off  period=1  dbl_ovrd=off
  sin0 : Outport
  sin1 : Outport  Port=2
  sin2 : Outport  Port=3
  sin3 : Outport  Port=4
  cos0 : Outport  Port=5
  cos1 : Outport  Port=6
  cos2 : Outport  Port=7
  cos3 : Outport  Port=8
  sync_out : Outport  Port=9
  wires:
  Convert6/1 -> Slice3/1
  Slice2/1 -> AddSub1/1
  Slice1/1 -> AddSub/1
  Slice8/1 -> AddSub4/2
  Convert4/1 -> Delay7/1, AddSub3/2, AddSub1/2, AddSub/2
  phase/1 -> Slice8/1
  AddSub4/1 -> Convert4/1
  Slice4/1 -> AddSub4/1
  SineCosine/2 -> cos0/1
  SineCosine/1 -> sin0/1
  SineCosine3/2 -> cos3/1
  SineCosine3/1 -> sin3/1
  SineCosine2/2 -> cos2/1
  SineCosine2/1 -> sin2/1
  SineCosine1/2 -> cos1/1
  SineCosine1/1 -> sin1/1
  Delay2/1 -> sync_out/1, Gateway Out4/1
  Delay7/1 -> Gateway Out/1, SineCosine/1, Gateway Out5/1
  sync_in/1 -> Delay2/1, Accumulator/2
  AddSub2/1 -> Convert6/1
  Shift1/1 -> Slice2/1
  Shift/1 -> AddSub2/2, Slice1/1
  AddSub3/1 -> Convert3/1
  AddSub1/1 -> Convert2/1
  AddSub/1 -> Convert1/1
  step/1 -> Shift/1, AddSub2/1, Shift1/1, Accumulator/1
  Accumulator/1 -> Slice4/1
  Convert1/1 -> Gateway Out1/1, SineCosine1/1, Gateway Out6/1
  Convert2/1 -> Gateway Out2/1, SineCosine2/1, Gateway Out7/1
  Convert3/1 -> SineCosine3/1, Gateway Out3/1, Gateway Out8/1
  Gateway Out/1 -> Scope/1
  Gateway Out1/1 -> Scope/2
  Gateway Out2/1 -> Scope/3
  Gateway Out3/1 -> Scope/4
  Slice3/1 -> AddSub3/1
  Multiport Switch/1 -> Scope3/1
  Gateway Out4/1 -> Scope3/2
  Counter Free-Running/1 -> Multiport Switch/1
  Gateway Out5/1 -> Multiport Switch/2
  Gateway Out6/1 -> Multiport Switch/3
  Gateway Out7/1 -> Multiport Switch/4
  Gateway Out8/1 -> Multiport Switch/5

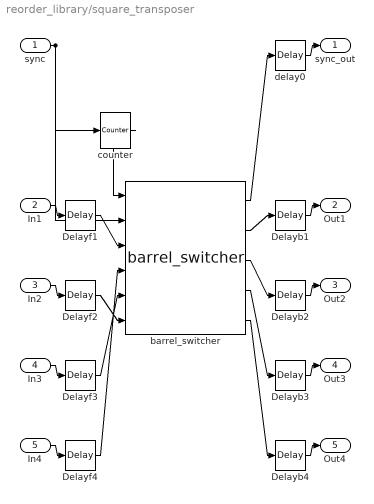
== system reorder_library/square_transposer ==
  sync : Inport  Port=1  LatchInput=off
  In1 : Inport  Port=2  LatchInput=off
  In2 : Inport  Port=3  LatchInput=off
  In3 : Inport  Port=4  LatchInput=off
  In4 : Inport  Port=5  LatchInput=off
  Delayb1 : xbsIndex_r3/Delay  latency=3  reg_retiming=off  explicit_period=off  period=1  en=off  accept_only_valid=off  init_zero=on  dbl_ovrd=off  show_param=off
      settings: xl_area=[0, 0, 0, 0, 0, 0, 0]
  Delayb2 : xbsIndex_r3/Delay  latency=2  reg_retiming=off  explicit_period=off  period=1  en=off  accept_only_valid=off  init_zero=on  dbl_ovrd=off  show_param=off
      settings: xl_area=[0, 0, 0, 0, 0, 0, 0]
  Delayb3 : xbsIndex_r3/Delay  latency=1  reg_retiming=off  explicit_period=off  period=1  en=off  accept_only_valid=off  init_zero=on  dbl_ovrd=off  show_param=off
      settings: xl_area=[0, 0, 0, 0, 0, 0, 0]
  Delayb4 : xbsIndex_r3/Delay  latency=0  reg_retiming=off  explicit_period=off  period=1  en=off  accept_only_valid=off  init_zero=on  dbl_ovrd=off  show_param=off
      settings: xl_area=[0, 0, 0, 0, 0, 0, 0]
  Delayf1 : xbsIndex_r3/Delay  latency=0  reg_retiming=off  explicit_period=off  period=1  en=off  accept_only_valid=off  init_zero=on  dbl_ovrd=off  show_param=off
      settings: xl_area=[0, 0, 0, 0, 0, 0, 0]
  Delayf2 : xbsIndex_r3/Delay  latency=1  reg_retiming=off  explicit_period=off  period=1  en=off  accept_only_valid=off  init_zero=on  dbl_ovrd=off  show_param=off
      settings: xl_area=[0, 0, 0, 0, 0, 0, 0]
  Delayf3 : xbsIndex_r3/Delay  latency=2  reg_retiming=off  explicit_period=off  period=1  en=off  accept_only_valid=off  init_zero=on  dbl_ovrd=off  show_param=off
      settings: xl_area=[0, 0, 0, 0, 0, 0, 0]
  Delayf4 : xbsIndex_r3/Delay  latency=3  reg_retiming=off  explicit_period=off  period=1  en=off  accept_only_valid=off  init_zero=on  dbl_ovrd=off  show_param=off
      settings: xl_area=[0, 0, 0, 0, 0, 0, 0]
  barrel_switcher : reorder_library/barrel_switcher  n_inputs=n_inputs
  counter : xbsIndex_r3/Counter  cnt_type=Free Running  n_bits=n_inputs  bin_pt=0  arith_type=Unsigned  start_count=0  cnt_to=Inf  cnt_by_val=1  operation=Down  explicit_period=off  period=1  load_pin=off  rst=on  en=off  dbl_ovrd=off  show_param=off  use_rpm=on  gen_core=off
      settings: xl_area=[0, 0, 0, 0, 0, 0, 0]
  delay0 : xbsIndex_r3/Delay  latency=2^n_inputs - 1  reg_retiming=off  explicit_period=off  period=1  en=off  accept_only_valid=off  init_zero=on  dbl_ovrd=off  show_param=off
      settings: xl_area=[0, 0, 0, 0, 0, 0, 0]
  sync_out : Outport
  Out1 : Outport  Port=2
  Out2 : Outport  Port=3
  Out3 : Outport  Port=4
  Out4 : Outport  Port=5
  wires:
  sync/1 -> counter/1, barrel_switcher/2
  counter/1 -> barrel_switcher/1
  barrel_switcher/1 -> delay0/1
  delay0/1 -> sync_out/1
  In1/1 -> Delayf1/1
  Delayf1/1 -> barrel_switcher/3
  barrel_switcher/2 -> Delayb1/1
  Delayb1/1 -> Out1/1
  In2/1 -> Delayf2/1
  Delayf2/1 -> barrel_switcher/6
  barrel_switcher/3 -> Delayb2/1
  Delayb2/1 -> Out2/1
  In3/1 -> Delayf3/1
  Delayf3/1 -> barrel_switcher/5
  barrel_switcher/4 -> Delayb3/1
  Delayb3/1 -> Out3/1
  In4/1 -> Delayf4/1
  Delayf4/1 -> barrel_switcher/4
  barrel_switcher/5 -> Delayb4/1
  Delayb4/1 -> Out4/1

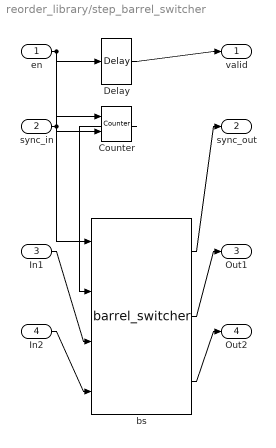
== system reorder_library/step_barrel_switcher ==
  en : Inport  Port=1  LatchInput=off
  sync_in : Inport  Port=2  LatchInput=off
  In1 : Inport  Port=3  LatchInput=off
  In2 : Inport  Port=4  LatchInput=off
  Counter : xbsIndex_r3/Counter  cnt_type=Free Running  n_bits=n_inputs  bin_pt=0  arith_type=Unsigned  start_count=0  cnt_to=Inf  cnt_by_val=1  operation=Up  explicit_period=off  period=1  load_pin=off  rst=on  en=on  dbl_ovrd=off  show_param=off  use_rpm=on  gen_core=off
      settings: xl_area=[0, 0, 0, 0, 0, 0, 0]
  Delay : xbsIndex_r3/Delay  latency=2  reg_retiming=off  explicit_period=off  period=1  en=off  accept_only_valid=off  init_zero=on  dbl_ovrd=off  show_param=off
      settings: xl_area=[0, 0, 0, 0, 0, 0, 0]
  bs : reorder_library/barrel_switcher  n_inputs=1
  valid : Outport
  sync_out : Outport  Port=2
  Out1 : Outport  Port=3
  Out2 : Outport  Port=4
  wires:
  en/1 -> Delay/1, Counter/2
  Delay/1 -> valid/1
  sync_in/1 -> Counter/1, bs/1
  Counter/1 -> bs/2
  bs/1 -> sync_out/1
  In1/1 -> bs/3
  bs/2 -> Out1/1
  In2/1 -> bs/4
  bs/3 -> Out2/1

== system reorder_library/dbuf_transpose_sram/addrMaker ==
  counter : Inport  Port=1  LatchInput=off
  Concat : xbsIndex_r3/Concat  num_inputs=2  explicit_period=off  period=1  dbl_ovrd=off
  Slice : xbsIndex_r3/Slice  mode=Lower Bit Location + Width  nbits=log2(numSpecs)  bit1=0  base1=MSB of Input  bit0=0  base0=LSB of Input  boolean_output=off  explicit_period=off  period=1  dbl_ovrd=off
  Slice1 : xbsIndex_r3/Slice  mode=Upper Bit Location + Width  nbits=log2(length)  bit1=0  base1=MSB of Input  bit0=0  base0=LSB of Input  boolean_output=off  explicit_period=off  period=1  dbl_ovrd=off
  writeAddr : Outport
  readAddr : Outport  Port=2
  wires:
  Concat/1 -> readAddr/1
  Slice1/1 -> Concat/2
  Slice/1 -> Concat/1
  counter/1 -> Slice1/1, Slice/1, writeAddr/1
